simulink model "LLC_Controller"  (R2022b)
settings: Solver=FixedStepDiscrete  StartTime=0.0  StopTime=Inf  FixedStep=(20e-6)  RelTol=1e-3  EnableMultiTasking=on
undefined symbols (not defined in the file): GPTRIP1SEL, GPTRIP2SEL, SCI_A_Transmit, SCI_A_Transmit_Current_Suffix, SCI_A_Transmit_Duty_Suffix, SCI_A_Transmit_Freq_Suffix, SCI_A_Transmit_NewVRegPoint_Suffix, SCI_A_Transmit_OCPFlag_Suffix, SCI_A_Transmit_OVPFlag_Suffix, SCI_A_Transmit_PFC_Suffix, SCI_A_Transmit_SS_Suffix, SCI_A_Transmit_TBPHS_Suffix, SCI_A_Transmit_VADC_Suffix, SCI_A_Transmit_VAvg_Suffix, SCI_A_Transmit_VBAT_Suffix, SCI_A_Transmit_VBATRef_Suffix, SCI_A_Transmit_Vo_Suffix, TZ1, TZ2
libraries: c280xlib x16, c28003xlib x13, c2802xlib x8, simulink x7, c2837xDlib x3, c2000lib x1
(part 2 of 2)

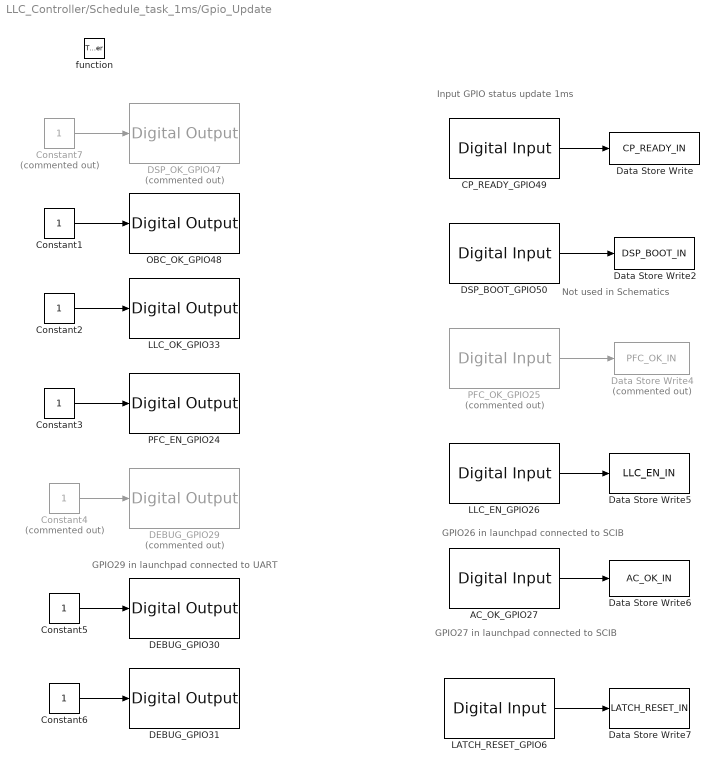
== system LLC_Controller/Schedule_task_1ms/Gpio_Update ==
  note: Not used in Schematics
  note: GPIO29 in launchpad connected to UART
  note: GPIO26 in launchpad connected to SCIB
  note: GPIO27 in launchpad connected to SCIB
  note: Input GPIO status update 1ms
  function : TriggerPort  TriggerType=function-call  VariantControl=(inherit)
  AC_OK_GPIO27 : c28003xlib/Digital Input  GPIO_Number=GPIO24~GPIO31  GPIO_Bit0=off  GPIO_Bit1=off  GPIO_Bit2=off  GPIO_Bit3=on  GPIO_Bit4=off  GPIO_Bit5=off  GPIO_Bit6=off  GPIO_Bit7=off  sampleTime=-1  dataType=auto  GPIO_Bit0_Qualification=Sync to SYSCLKOUT  GPIO_Bit1_Qualification=Sync to SYSCLKOUT  GPIO_Bit2_Qualification=Sync to SYSCLKOUT  GPIO_Bit3_Qualification=Sync to SYSCLKOUT  GPIO_Bit4_Qualification=Sync to SYSCLKOUT  GPIO_Bit5_Qualification=Sync to SYSCLKOUT  GPIO_Bit6_Qualification=Sync to SYSCLKOUT  GPIO_Bit7_Qualification=Sync to SYSCLKOUT  Qualification_Period=-1
  CP_READY_GPIO49 : c28003xlib/Digital Input  GPIO_Number=GPIO48~GPIO55  GPIO_Bit0=off  GPIO_Bit1=on  GPIO_Bit2=off  GPIO_Bit3=off  GPIO_Bit4=off  GPIO_Bit5=off  GPIO_Bit6=off  GPIO_Bit7=off  sampleTime=-1  dataType=auto  GPIO_Bit0_Qualification=Sync to SYSCLKOUT  GPIO_Bit1_Qualification=Sync to SYSCLKOUT  GPIO_Bit2_Qualification=Sync to SYSCLKOUT  GPIO_Bit3_Qualification=Sync to SYSCLKOUT  GPIO_Bit4_Qualification=Sync to SYSCLKOUT  GPIO_Bit5_Qualification=Sync to SYSCLKOUT  GPIO_Bit6_Qualification=Sync to SYSCLKOUT  GPIO_Bit7_Qualification=Sync to SYSCLKOUT  Qualification_Period=-1
  Constant{1..3,5..6} (5 alike) : Constant  OutDataTypeStr=boolean  SampleTime=-1
  Constant4 : Constant  Commented=on  OutDataTypeStr=boolean  SampleTime=-1
  Constant7 : Constant  Commented=on  OutDataTypeStr=boolean  SampleTime=-1
  DEBUG_GPIO29 : c28003xlib/Digital Output  Commented=on  GPIO_Number=GPIO24~GPIO31  GPIO_Bit0=off  GPIO_BIT0_Toggle=on  GPIO_Bit1=off  GPIO_BIT1_Toggle=on  GPIO_Bit2=off  GPIO_BIT2_Toggle=off  GPIO_Bit3=off  GPIO_BIT3_Toggle=off  GPIO_Bit4=off  GPIO_BIT4_Toggle=on  GPIO_Bit5=on  GPIO_BIT5_Toggle=on  GPIO_Bit6=off  GPIO_BIT6_Toggle=on  GPIO_Bit7=off  GPIO_BIT7_Toggle=on
  DEBUG_GPIO30 : c28003xlib/Digital Output  GPIO_Number=GPIO24~GPIO31  GPIO_Bit0=off  GPIO_BIT0_Toggle=on  GPIO_Bit1=off  GPIO_BIT1_Toggle=on  GPIO_Bit2=off  GPIO_BIT2_Toggle=off  GPIO_Bit3=off  GPIO_BIT3_Toggle=off  GPIO_Bit4=off  GPIO_BIT4_Toggle=on  GPIO_Bit5=off  GPIO_BIT5_Toggle=on  GPIO_Bit6=on  GPIO_BIT6_Toggle=on  GPIO_Bit7=off  GPIO_BIT7_Toggle=on
  DEBUG_GPIO31 : c28003xlib/Digital Output  GPIO_Number=GPIO24~GPIO31  GPIO_Bit0=off  GPIO_BIT0_Toggle=on  GPIO_Bit1=off  GPIO_BIT1_Toggle=on  GPIO_Bit2=off  GPIO_BIT2_Toggle=off  GPIO_Bit3=off  GPIO_BIT3_Toggle=off  GPIO_Bit4=off  GPIO_BIT4_Toggle=on  GPIO_Bit5=off  GPIO_BIT5_Toggle=on  GPIO_Bit6=off  GPIO_BIT6_Toggle=on  GPIO_Bit7=on  GPIO_BIT7_Toggle=on
  DSP_BOOT_GPIO50 : c28003xlib/Digital Input  GPIO_Number=GPIO48~GPIO55  GPIO_Bit0=off  GPIO_Bit1=off  GPIO_Bit2=on  GPIO_Bit3=off  GPIO_Bit4=off  GPIO_Bit5=off  GPIO_Bit6=off  GPIO_Bit7=off  sampleTime=-1  dataType=auto  GPIO_Bit0_Qualification=Sync to SYSCLKOUT  GPIO_Bit1_Qualification=Sync to SYSCLKOUT  GPIO_Bit2_Qualification=Sync to SYSCLKOUT  GPIO_Bit3_Qualification=Sync to SYSCLKOUT  GPIO_Bit4_Qualification=Sync to SYSCLKOUT  GPIO_Bit5_Qualification=Sync to SYSCLKOUT  GPIO_Bit6_Qualification=Sync to SYSCLKOUT  GPIO_Bit7_Qualification=Sync to SYSCLKOUT  Qualification_Period=-1
  DSP_OK_GPIO47 : c28003xlib/Digital Output  Commented=on  GPIO_Number=GPIO40~GPIO47  GPIO_Bit0=off  GPIO_BIT0_Toggle=on  GPIO_Bit1=off  GPIO_BIT1_Toggle=off  GPIO_Bit2=off  GPIO_BIT2_Toggle=off  GPIO_Bit3=off  GPIO_BIT3_Toggle=off  GPIO_Bit4=off  GPIO_BIT4_Toggle=on  GPIO_Bit5=off  GPIO_BIT5_Toggle=off  GPIO_Bit6=off  GPIO_BIT6_Toggle=off  GPIO_Bit7=on  GPIO_BIT7_Toggle=off
  Data Store Write : DataStoreWrite  DataStoreName=CP_READY_IN  IndexOptions=Index vector (dialog)  Indices=1  OutputSizes=1
  Data Store Write2 : DataStoreWrite  DataStoreName=DSP_BOOT_IN  IndexOptions=Index vector (dialog)  Indices=1  OutputSizes=1
  Data Store Write4 : DataStoreWrite  Commented=on  DataStoreName=PFC_OK_IN  IndexOptions=Index vector (dialog)  Indices=1  OutputSizes=1
  Data Store Write5 : DataStoreWrite  DataStoreName=LLC_EN_IN  IndexOptions=Index vector (dialog)  Indices=1  OutputSizes=1
  Data Store Write6 : DataStoreWrite  DataStoreName=AC_OK_IN  IndexOptions=Index vector (dialog)  Indices=1  OutputSizes=1
  Data Store Write7 : DataStoreWrite  DataStoreName=LATCH_RESET_IN  IndexOptions=Index vector (dialog)  Indices=1  OutputSizes=1
  LATCH_RESET_GPIO6 : c28003xlib/Digital Input  GPIO_Number=GPIO0~GPIO7  GPIO_Bit0=off  GPIO_Bit1=off  GPIO_Bit2=off  GPIO_Bit3=off  GPIO_Bit4=off  GPIO_Bit5=off  GPIO_Bit6=on  GPIO_Bit7=off  sampleTime=-1  dataType=auto  GPIO_Bit0_Qualification=Sync to SYSCLKOUT  GPIO_Bit1_Qualification=Sync to SYSCLKOUT  GPIO_Bit2_Qualification=Sync to SYSCLKOUT  GPIO_Bit3_Qualification=Sync to SYSCLKOUT  GPIO_Bit4_Qualification=Sync to SYSCLKOUT  GPIO_Bit5_Qualification=Sync to SYSCLKOUT  GPIO_Bit6_Qualification=Sync to SYSCLKOUT  GPIO_Bit7_Qualification=Sync to SYSCLKOUT  Qualification_Period=-1
  LLC_EN_GPIO26 : c28003xlib/Digital Input  GPIO_Number=GPIO24~GPIO31  GPIO_Bit0=off  GPIO_Bit1=off  GPIO_Bit2=on  GPIO_Bit3=off  GPIO_Bit4=off  GPIO_Bit5=off  GPIO_Bit6=off  GPIO_Bit7=off  sampleTime=-1  dataType=auto  GPIO_Bit0_Qualification=Sync to SYSCLKOUT  GPIO_Bit1_Qualification=Sync to SYSCLKOUT  GPIO_Bit2_Qualification=Sync to SYSCLKOUT  GPIO_Bit3_Qualification=Sync to SYSCLKOUT  GPIO_Bit4_Qualification=Sync to SYSCLKOUT  GPIO_Bit5_Qualification=Sync to SYSCLKOUT  GPIO_Bit6_Qualification=Sync to SYSCLKOUT  GPIO_Bit7_Qualification=Sync to SYSCLKOUT  Qualification_Period=-1
  LLC_OK_GPIO33 : c28003xlib/Digital Output  GPIO_Number=GPIO32~GPIO39  GPIO_Bit0=off  GPIO_BIT0_Toggle=off  GPIO_Bit1=on  GPIO_BIT1_Toggle=on  GPIO_Bit2=off  GPIO_BIT2_Toggle=off  GPIO_Bit3=off  GPIO_BIT3_Toggle=off  GPIO_Bit4=off  GPIO_BIT4_Toggle=on  GPIO_Bit5=off  GPIO_BIT5_Toggle=off  GPIO_Bit6=off  GPIO_BIT6_Toggle=off  GPIO_Bit7=off  GPIO_BIT7_Toggle=off
  OBC_OK_GPIO48 : c28003xlib/Digital Output  GPIO_Number=GPIO48~GPIO55  GPIO_Bit0=on  GPIO_BIT0_Toggle=on  GPIO_Bit1=off  GPIO_BIT1_Toggle=off  GPIO_Bit2=off  GPIO_BIT2_Toggle=off  GPIO_Bit3=off  GPIO_BIT3_Toggle=off  GPIO_Bit4=off  GPIO_BIT4_Toggle=on  GPIO_Bit5=off  GPIO_BIT5_Toggle=off  GPIO_Bit6=off  GPIO_BIT6_Toggle=off  GPIO_Bit7=off  GPIO_BIT7_Toggle=off
  PFC_EN_GPIO24 : c28003xlib/Digital Output  GPIO_Number=GPIO24~GPIO31  GPIO_Bit0=on  GPIO_BIT0_Toggle=on  GPIO_Bit1=off  GPIO_BIT1_Toggle=on  GPIO_Bit2=off  GPIO_BIT2_Toggle=off  GPIO_Bit3=off  GPIO_BIT3_Toggle=off  GPIO_Bit4=off  GPIO_BIT4_Toggle=on  GPIO_Bit5=off  GPIO_BIT5_Toggle=off  GPIO_Bit6=off  GPIO_BIT6_Toggle=off  GPIO_Bit7=off  GPIO_BIT7_Toggle=off
  PFC_OK_GPIO25 : c28003xlib/Digital Input  Commented=on  GPIO_Number=GPIO24~GPIO31  GPIO_Bit0=off  GPIO_Bit1=on  GPIO_Bit2=off  GPIO_Bit3=off  GPIO_Bit4=off  GPIO_Bit5=off  GPIO_Bit6=off  GPIO_Bit7=off  sampleTime=-1  dataType=auto  GPIO_Bit0_Qualification=Sync to SYSCLKOUT  GPIO_Bit1_Qualification=Sync to SYSCLKOUT  GPIO_Bit2_Qualification=Sync to SYSCLKOUT  GPIO_Bit3_Qualification=Sync to SYSCLKOUT  GPIO_Bit4_Qualification=Sync to SYSCLKOUT  GPIO_Bit5_Qualification=Sync to SYSCLKOUT  GPIO_Bit6_Qualification=Sync to SYSCLKOUT  GPIO_Bit7_Qualification=Sync to SYSCLKOUT  Qualification_Period=-1
  wires:
  Constant1/1 -> OBC_OK_GPIO48/1
  Constant2/1 -> LLC_OK_GPIO33/1
  AC_OK_GPIO27/1 -> Data Store Write6/1
  LATCH_RESET_GPIO6/1 -> Data Store Write7/1
  PFC_OK_GPIO25/1 -> Data Store Write4/1
  Constant4/1 -> DEBUG_GPIO29/1
  CP_READY_GPIO49/1 -> Data Store Write/1
  LLC_EN_GPIO26/1 -> Data Store Write5/1
  DSP_BOOT_GPIO50/1 -> Data Store Write2/1
  Constant6/1 -> DEBUG_GPIO31/1
  Constant3/1 -> PFC_EN_GPIO24/1
  Constant5/1 -> DEBUG_GPIO30/1
  Constant7/1 -> DSP_OK_GPIO47/1

== system LLC_Controller/State_Machine/LLC_STATEFLOW/SSvoltage ==
  f : TriggerPort  TriggerType=function-call  VariantControl=(inherit)
      settings: CopyFcn=Stateflow.SLINSF.SimulinkMan.removeBlockPreDeleteFcn  PreDeleteFcn=Stateflow.SLINSF.SimulinkMan.unsafePredeleteFcn
  Chart1 : Stateflow chart  TreatAsAtomicUnit=on
  Constant1 : Constant  OutDataTypeStr=double  SampleTime=Inf
  wires:
  Constant1/1 -> Chart1/1(VBAT_Ref)

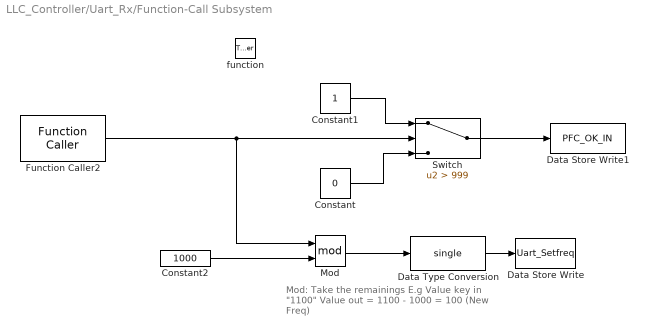
== system LLC_Controller/Uart_Rx/Function-Call Subsystem ==
  note: Mod: Take the remainings
      | E.g
      | Value key in "1100"
      | Value out = 1100 - 1000 = 100 (New Freq)
  function : TriggerPort  TriggerType=function-call  VariantControl=(inherit)
  Constant : Constant  Value=0
  Constant1 : Constant
  Constant2 : Constant  Value=1000
  Data Store Write : DataStoreWrite  DataStoreName=Uart_Setfreq  IndexOptions=Index vector (dialog)  Indices=1  OutputSizes=1
  Data Store Write1 : DataStoreWrite  DataStoreName=PFC_OK_IN  IndexOptions=Index vector (dialog)  Indices=1  OutputSizes=1
  Data Type Conversion : DataTypeConversion  OutDataTypeStr=single  SaturateOnIntegerOverflow=off  RndMeth=Floor
  Function Caller2 : FunctionCaller  FunctionPrototype=y = SCI_Receive()  InputArgumentSpecifications=<Enter example>  OutputArgumentSpecifications=<Enter example>
  Mod : Math  Operator=mod
  Switch : Switch  Criteria=u2 > Threshold  Threshold=999  SaturateOnIntegerOverflow=off  InputSameDT=off
  wires:
  Switch/1 -> Data Store Write1/1
  Function Caller2/1 -> Mod/1, Switch/2
  Constant/1 -> Switch/3
  Constant1/1 -> Switch/1
  Mod/1 -> Data Type Conversion/1
  Constant2/1 -> Mod/2
  Data Type Conversion/1 -> Data Store Write/1

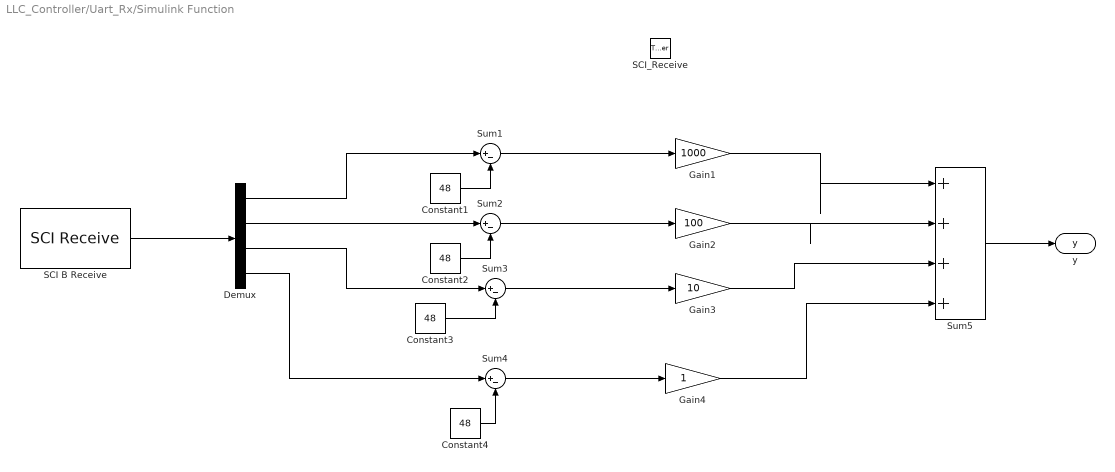
== system LLC_Controller/Uart_Rx/Simulink Function ==
  SCI_Receive : TriggerPort  TriggerType=function-call  IsSimulinkFunction=on  FunctionName=SCI_Receive  FunctionVisibility=scoped  VariantControl=(inherit)
  Constant{1..4} (4 alike) : Constant  Value=48
  Demux : Demux
  Gain1 : Gain  Gain=1000
  Gain2 : Gain  Gain=100
  Gain3 : Gain  Gain=10
  Gain4 : Gain
  SCI B Receive : c280xlib/SCI Receive  Priority=2  sciModule=A  dataHead=''  headerCheckMaxCount=16  dataTail=''  dataType=uint8  dataLenOptions=Length via dialog  dataDim=4  maxDataLength=100  initValue=0  errOption=Output custom value  errValue=0  sampleTime=-1  blockingMode=on  timeOut=0.01944  outputStatus=off
      settings: LibrarySourceBlock=c2806xlib/SCI Receive
  Sum{1..4} (4 alike) : Sum  Inputs=|+-
  Sum5 : Sum  Inputs=|++++  AccumDataTypeStr=double  OutDataTypeStr=double
  y : ArgOut  DisableCoverage=on  ArgumentName=y
  wires:
  Gain2/1 -> Sum5/2
  Gain3/1 -> Sum5/3
  Constant3/1 -> Sum3/2
  Sum4/1 -> Gain4/1
  Constant2/1 -> Sum2/2
  Sum2/1 -> Gain2/1
  SCI B Receive/1 -> Demux/1
  Constant4/1 -> Sum4/2
  Sum3/1 -> Gain3/1
  Sum5/1 -> y/1
  Demux/4 -> Sum4/1
  Demux/3 -> Sum3/1
  Demux/2 -> Sum2/1
  Constant1/1 -> Sum1/2
  Demux/1 -> Sum1/1
  Gain4/1 -> Sum5/4
  Gain1/1 -> Sum5/1
  Sum1/1 -> Gain1/1

== system LLC_Controller/LLC Control/LLC_On_Off_Control/Subsystem_llc_off ==
  Action Port : ActionPort  ActionPortLabel=else
  Constant : Constant  OutDataTypeStr=boolean
  Data Store Write : DataStoreWrite  DataStoreName=LLC_Clr_tz  IndexOptions=Index vector (dialog)  Indices=1  OutputSizes=1
  PWM_LLC_OFF : Subsystem  mask(System Outputs){ShowInLibBrowser=0}
      mask prompts: ShowInLibBrowser "Simulink:masks:CustCodeMaskParam1_MP"
      settings: CopyFcn=cccopyfcn(gcb)  OpenFcn=ccopenfcn('System Outputs Function')
      mask Help: eval('feval(''rtwprivate'',''rtwhelpview'',''rtw_sys_outputs_block'')');
      mask DialogControl ShowInLibBrowser Prompt: Mask Parameter 1:
      mask Display: disp('System\nOutputs');
  wires:
  Constant/1 -> Data Store Write/1

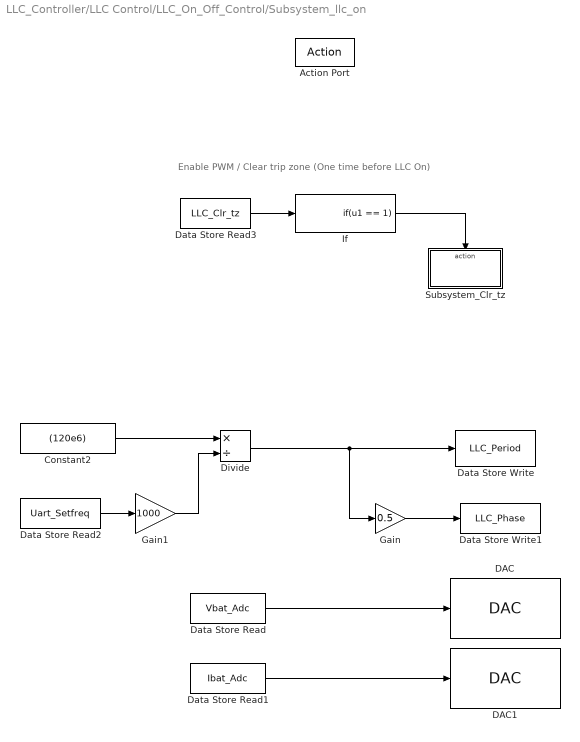
== system LLC_Controller/LLC Control/LLC_On_Off_Control/Subsystem_llc_on ==
  note: Enable PWM / Clear trip zone (One time before LLC On)
  Action Port : ActionPort  ActionPortLabel=if(u1 == 1)
  Constant2 : Constant  Value=(120e6)  OutDataTypeStr=single  SampleTime=-1
  DAC : c2837xDlib/DAC  channel=A  saturate=on
      settings: LibrarySourceBlock=c28003xlib/DAC
  DAC1 : c2837xDlib/DAC  channel=B  saturate=on
      settings: LibrarySourceBlock=c28003xlib/DAC
  Data Store Read : DataStoreRead  DataStoreName=Vbat_Adc  IndexOptions=Index vector (dialog)  Indices=1  OutputSizes=1
  Data Store Read1 : DataStoreRead  DataStoreName=Ibat_Adc  IndexOptions=Index vector (dialog)  Indices=1  OutputSizes=1
  Data Store Read2 : DataStoreRead  DataStoreName=Uart_Setfreq  IndexOptions=Index vector (dialog)  Indices=1  OutputSizes=1
  Data Store Read3 : DataStoreRead  DataStoreName=LLC_Clr_tz  IndexOptions=Index vector (dialog)  Indices=1  OutputSizes=1
  Data Store Write : DataStoreWrite  DataStoreName=LLC_Period  IndexOptions=Index vector (dialog)  Indices=1  OutputSizes=1
  Data Store Write1 : DataStoreWrite  DataStoreName=LLC_Phase  IndexOptions=Index vector (dialog)  Indices=1  OutputSizes=1
  Divide : Product  Inputs=*/  OutDataTypeStr=single
  Gain : Gain  Gain=0.5  OutDataTypeStr=single
  Gain1 : Gain  Gain=1000  OutDataTypeStr=single
  If : If  IfExpression=u1 == 1  ShowElse=off
  Subsystem_Clr_tz : Subsystem  TreatAsAtomicUnit=on
  wires:
  If/1 -> Subsystem_Clr_tz/Action
  Data Store Read3/1 -> If/1
  Divide/1 -> Gain/1, Data Store Write/1
  Gain/1 -> Data Store Write1/1
  Data Store Read/1 -> DAC/1
  Data Store Read1/1 -> DAC1/1
  Constant2/1 -> Divide/1
  Gain1/1 -> Divide/2
  Data Store Read2/1 -> Gain1/1

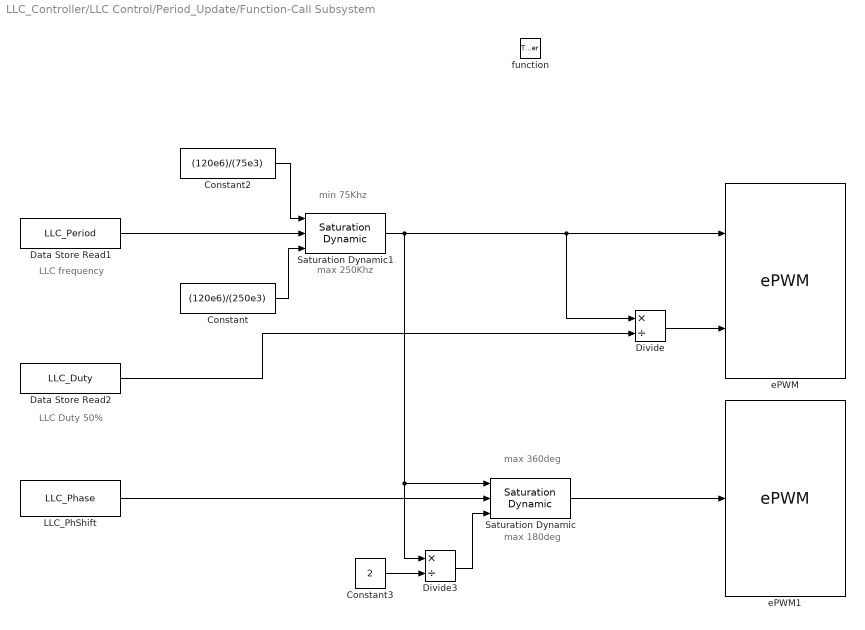
== system LLC_Controller/LLC Control/Period_Update/Function-Call Subsystem ==
  note: LLC frequency
  note: LLC Duty 50%
  note: max 180deg
  note: max 360deg
  note: min 75Khz
  note: max 250Khz
  function : TriggerPort  TriggerType=function-call  VariantControl=(inherit)
  Constant : Constant  Value=(120e6)/(250e3)  OutDataTypeStr=single  SampleTime=-1
  Constant2 : Constant  Value=(120e6)/(75e3)  OutDataTypeStr=single  SampleTime=-1
  Constant3 : Constant  Value=2  OutDataTypeStr=single  SampleTime=-1
  Data Store Read1 : DataStoreRead  DataStoreName=LLC_Period  IndexOptions=Index vector (dialog)  Indices=1  OutputSizes=1
  Data Store Read2 : DataStoreRead  DataStoreName=LLC_Duty  IndexOptions=Index vector (dialog)  Indices=1  OutputSizes=1
  Divide : Product  Inputs=*/
  Divide3 : Product  Inputs=*/
  LLC_PhShift : DataStoreRead  DataStoreName=LLC_Phase  IndexOptions=Index vector (dialog)  Indices=1  OutputSizes=1
  Saturation Dynamic : simulink/Discontinuities/Saturation Dynamic  OutMin=[]  OutMax=[]  OutDataTypeStr=Inherit: Same as second input  OutDataType=fixdt(1, 16)  OutScaling=2^-10  DoSatur=off
  Saturation Dynamic1 : simulink/Discontinuities/Saturation Dynamic  OutMin=[]  OutMax=[]  OutDataTypeStr=Inherit: Same as second input  OutDataType=fixdt(1, 16)  OutScaling=2^-10  DoSatur=off
  ePWM : c2802xlib/ePWM  PwmType=C2000_Type4_F28002x  useModule=ePWM5  ePWMxLINKTBPRD=Not Linked  periodUnits=Clock cycles  timerSource=Input port  timerPeriod_clk=600  timerPeriod_sec=0.0001  tbshadow=Counter equals to zero  countingMode=Up  phaseActiveEnable=Disable  phaseDirection=Count down after sync  phaseActive=0  synchronizationEnable=off  dcaevt1Sync=off  dcbevt1Sync=off  synchronizationOption=Counter equals to zero (CTR=Zero)  dcbevt1SyncOut=off  dcaevt1SyncOut=off  cmpdSyncOut=off  cmpcSyncOut=off  cmpbSyncOut=off  zeroSyncOut=on  swfSyncOut=off  perSynchronizationOption=Counter equals to period (CTR=PRD)  clockPrescale=1  HSclockPrescale=1  enswap=off  ePWMxAStatus=on  ePWMxAactionLogic1=Set  ePWMxAactionLogic2=Do nothing  ePWMxAactionLogic3=Clear  ePWMxAactionLogic4=Do nothing  ePWMxAactionLogic5=Do nothing  ePWMxAactionLogic6=Do nothing  ePWMxACSFenable=off  ePWMxACSFvalue=Forcing disable  ePWMxASFreload=Zero  ePWMxBStatus=on  ePWMxBactionLogic1=Clear  ePWMxBactionLogic2=Do nothing  ePWMxBactionLogic3=Set  ePWMxBactionLogic4=Do nothing  ePWMxBactionLogic5=Do nothing  ePWMxBactionLogic6=Set  ePWMxBCSFenable=off  ePWMxBCSFvalue=Forcing disable  ePWMxBSFreload=Zero  ePWNxBOutWay=off  ePWMxLINKCMPA=Not Linked  CMPAUnits=Clock cycles  CMPASource=Input port  CMPAValue_per=50  CMPAValue_clk=298  enCMPAshadow=Counter equals to zero (CTR=Zero)  ePWMxLINKCMPB=Not Linked  CMPBUnits=Clock cycles  CMPBSource=Specify via dialog  CMPBValue_per=50  CMPBValue_clk=0  enCMPBshadow=Counter equals to zero (CTR=Zero)  ePWMxLINKCMPC=Not Linked  CMPCUnits=Clock cycles  CMPCSource=Specify via dialog  CMPCValue_per=50  CMPCValue_clk=32000  enCMPCshadow=Counter equals to zero (CTR=Zero)  ePWMxLINKCMPD=Not Linked  CMPDUnits=Percentages  CMPDSource=Specify via dialog  CMPDValue_per=50  CMPDValue_clk=32000  enCMPDshadow=Counter equals to zero (CTR=Zero)  enableDBePWMxA=on  enableDBePWMxB=on  enhalfcycle=off  DBpolarity=Active high complementary (AHC)  DBedgeDelay=Positive  DBSource_ePWMxA=ePWMxA  DBSource_ePWMxB=ePWMxA  DBPeriodUnits=Seconds  DBperiodSource=Specify via dialog  REDperiod=0  FEDperiod=0  REDperiod_sec=250e-9  FEDperiod_sec=250e-9  LoadModeDBRED=Counter equals to zero (CTR=ZERO)  LoadModeDBFED=Counter equals to zero (CTR=ZERO)  adcstartModuleA=off  adcrequestEventA=First event  adcstartEventA=Counter equals to zero (CTR=Zero)  adcstartEventA_type2=Counter equals to zero (CTR=Zero)  adcstartModuleB=off  adcrequestEventB=First event  adcstartEventB=Counter equals to zero (CTR=Zero)  adcstartEventB_type2=Counter equals to zero (CTR=Zero)  intEn=off  intPrd=First event  intSel=Counter equals to zero (CTR=Zero)  intSel_type2=Counter equals to zero (CTR=Zero)  hrpe=off  enHRPWM=off  HRPWM_LoadMode=Counter equals to zero (CTR=ZERO)  HRPWM_CTLMode=Duty or Period control mode  HRPWM_EDGMode=Both edge  hrpeb=off  enHRPWMB=off  HRPWM_LoadModeB=Counter equals to zero (CTR=ZERO)  HRPWM_CTLModeB=Duty or Period control mode  HRPWM_EDGModeB=Both edge  enHRDBRED=off  enHRDBFED=off  enSFO=on  enautoconv=on  chopperEnable=off  chopperFrequency=1  chopperFirstwidth=1  chopperDuty=12.5%  tripZonesource=Specify via dialog  tzselOSHT1=off  tzselOSHT2=off  tzselOSHT3=off  tzselOSHDCAEV1=off  tzselOSHDCBEV1=off  tzselCBC1=off  tzselCBC2=off  tzselCBC3=off  tzselCBCDCAEV2=off  tzselCBCDCBEV2=off  tzselOSHT4=off  tzselOSHT5=off  tzselOSHT6=off  tzselCBC4=off  tzselCBC5=off  tzselCBC6=off  enTzOstIntr=off  enTzCbcIntr=off  enTzDCAEVT1Intr=off  enTzDCAEVT2Intr=off  enTzDCBEVT1Intr=off  enTzDCBEVT2Intr=off  ePWMxAforced=Low  ePWMxBforced=Low  DCAEVT1forced=No action  DCBEVT1forced=No action  DCAEVT2forced=No action  DCBEVT2forced=No action  dcah=Trip Zone 1 input (TZ1)  dcal=Trip Zone 1 input (TZ1)  dcbh=Trip Zone 1 input (TZ1)  dcbl=Trip Zone 1 input (TZ1)  dcah_type2=GPTRIP4SEL  dcal_type2=GPTRIP1SEL/(TZ1)  dcbh_type2=GPTRIP4SEL  dcbl_type2=GPTRIP2SEL/(TZ2)  gendcaevt1=DCAH=high and DCAL=don't care  gendcaevt2=Event disabled  gendcbevt1=DCBH=high and DCBL=don't care  gendcbevt2=Event disabled  dcaevt1src=DCAEVT1 with async  dcaevt2src=DCAEVT2 with sync  dcbevt1src=DCBEVT1 with async  dcbevt2src=DCBEVT2 with sync  pulsesel=Counter equals to zero (CTR=Zero)  blankinv=off  blankoffset=0  blankwidth=0  evsrcsel=Filtered version of DCAEVT1 (DCAEVT1FILT)  encape=off
  ePWM1 : c2802xlib/ePWM  PwmType=C2000_Type4_F28002x  useModule=ePWM7  ePWMxLINKTBPRD=ePWM5  periodUnits=Clock cycles  timerSource=Specify via dialog  timerPeriod_clk=600  timerPeriod_sec=0.0001  tbshadow=Counter equals to zero  countingMode=Up  phaseActiveEnable=Set counter to phase value specified via input port  phaseDirection=Count down after sync  phaseActive=0  synchronizationEnable=off  dcaevt1Sync=off  dcbevt1Sync=off  synchronizationOption=Counter equals to zero (CTR=Zero)  dcbevt1SyncOut=off  dcaevt1SyncOut=off  cmpdSyncOut=off  cmpcSyncOut=off  cmpbSyncOut=off  zeroSyncOut=on  swfSyncOut=off  perSynchronizationOption=Counter equals to zero (CTR=Zero)  clockPrescale=1  HSclockPrescale=1  enswap=off  ePWMxAStatus=on  ePWMxAactionLogic1=Set  ePWMxAactionLogic2=Do nothing  ePWMxAactionLogic3=Clear  ePWMxAactionLogic4=Do nothing  ePWMxAactionLogic5=Do nothing  ePWMxAactionLogic6=Do nothing  ePWMxACSFenable=off  ePWMxACSFvalue=Forcing disable  ePWMxASFreload=Zero  ePWMxBStatus=on  ePWMxBactionLogic1=Clear  ePWMxBactionLogic2=Do nothing  ePWMxBactionLogic3=Set  ePWMxBactionLogic4=Do nothing  ePWMxBactionLogic5=Do nothing  ePWMxBactionLogic6=Set  ePWMxBCSFenable=off  ePWMxBCSFvalue=Forcing disable  ePWMxBSFreload=Zero  ePWNxBOutWay=off  ePWMxLINKCMPA=ePWM5  CMPAUnits=Clock cycles  CMPASource=Specify via dialog  CMPAValue_per=50  CMPAValue_clk=298  enCMPAshadow=Counter equals to zero (CTR=Zero)  ePWMxLINKCMPB=Not Linked  CMPBUnits=Clock cycles  CMPBSource=Specify via dialog  CMPBValue_per=50  CMPBValue_clk=0  enCMPBshadow=Counter equals to zero (CTR=Zero)  ePWMxLINKCMPC=Not Linked  CMPCUnits=Clock cycles  CMPCSource=Specify via dialog  CMPCValue_per=50  CMPCValue_clk=32000  enCMPCshadow=Counter equals to zero (CTR=Zero)  ePWMxLINKCMPD=Not Linked  CMPDUnits=Percentages  CMPDSource=Specify via dialog  CMPDValue_per=50  CMPDValue_clk=32000  enCMPDshadow=Counter equals to zero (CTR=Zero)  enableDBePWMxA=on  enableDBePWMxB=on  enhalfcycle=off  DBpolarity=Active high complementary (AHC)  DBedgeDelay=Positive  DBSource_ePWMxA=ePWMxA  DBSource_ePWMxB=ePWMxA  DBPeriodUnits=Seconds  DBperiodSource=Specify via dialog  REDperiod=0  FEDperiod=0  REDperiod_sec=250e-9  FEDperiod_sec=250e-9  LoadModeDBRED=Counter equals to zero (CTR=ZERO)  LoadModeDBFED=Counter equals to zero (CTR=ZERO)  adcstartModuleA=off  adcrequestEventA=First event  adcstartEventA=Counter equals to zero (CTR=Zero)  adcstartEventA_type2=Counter equals to zero (CTR=Zero)  adcstartModuleB=off  adcrequestEventB=First event  adcstartEventB=Counter equals to zero (CTR=Zero)  adcstartEventB_type2=Counter equals to zero (CTR=Zero)  intEn=off  intPrd=First event  intSel=Counter equals to zero (CTR=Zero)  intSel_type2=Counter equals to zero (CTR=Zero)  hrpe=off  enHRPWM=off  HRPWM_LoadMode=Counter equals to period (CTR=PRD)  HRPWM_CTLMode=Duty or Period control mode  HRPWM_EDGMode=Both edge  hrpeb=off  enHRPWMB=off  HRPWM_LoadModeB=Counter equals to zero (CTR=ZERO)  HRPWM_CTLModeB=Duty or Period control mode  HRPWM_EDGModeB=Both edge  enHRDBRED=off  enHRDBFED=off  enSFO=on  enautoconv=on  chopperEnable=off  chopperFrequency=1  chopperFirstwidth=1  chopperDuty=12.5%  tripZonesource=Specify via dialog  tzselOSHT1=off  tzselOSHT2=off  tzselOSHT3=off  tzselOSHDCAEV1=off  tzselOSHDCBEV1=off  tzselCBC1=off  tzselCBC2=off  tzselCBC3=off  tzselCBCDCAEV2=off  tzselCBCDCBEV2=off  tzselOSHT4=off  tzselOSHT5=off  tzselOSHT6=off  tzselCBC4=off  tzselCBC5=off  tzselCBC6=off  enTzOstIntr=off  enTzCbcIntr=off  enTzDCAEVT1Intr=off  enTzDCAEVT2Intr=off  enTzDCBEVT1Intr=off  enTzDCBEVT2Intr=off  ePWMxAforced=Low  ePWMxBforced=Low  DCAEVT1forced=No action  DCBEVT1forced=No action  DCAEVT2forced=No action  DCBEVT2forced=No action  dcah=Trip Zone 1 input (TZ1)  dcal=Trip Zone 1 input (TZ1)  dcbh=Trip Zone 1 input (TZ1)  dcbl=Trip Zone 1 input (TZ1)  dcah_type2=GPTRIP4SEL  dcal_type2=GPTRIP2SEL/(TZ2)  dcbh_type2=GPTRIP4SEL  dcbl_type2=GPTRIP2SEL/(TZ2)  gendcaevt1=DCAH=high and DCAL=don't care  gendcaevt2=Event disabled  gendcbevt1=DCBH=high and DCBL=don't care  gendcbevt2=Event disabled  dcaevt1src=DCAEVT1 with async  dcaevt2src=DCAEVT2 with sync  dcbevt1src=DCBEVT1 with async  dcbevt2src=DCBEVT2 with sync  pulsesel=Counter equals to zero (CTR=Zero)  blankinv=off  blankoffset=0  blankwidth=0  evsrcsel=Filtered version of DCAEVT1 (DCAEVT1FILT)  encape=off
  wires:
  Saturation Dynamic/1 -> ePWM1/1
  Divide/1 -> ePWM/2
  Data Store Read2/1 -> Divide/2
  Constant/1 -> Saturation Dynamic1/3
  Saturation Dynamic1/1 -> Divide3/1, Saturation Dynamic/1, Divide/1, ePWM/1
  Constant2/1 -> Saturation Dynamic1/1
  Divide3/1 -> Saturation Dynamic/3
  Constant3/1 -> Divide3/2
  LLC_PhShift/1 -> Saturation Dynamic/2
  Data Store Read1/1 -> Saturation Dynamic1/2

== system LLC_Controller/LLC Control/Period_Update/Function-Call Subsystem1 ==
  function : TriggerPort  TriggerType=function-call  VariantControl=(inherit)
  PWM_UPDATE : Subsystem  mask(System Outputs){ShowInLibBrowser=0}
      mask prompts: ShowInLibBrowser "Simulink:masks:CustCodeMaskParam1_MP"
      settings: CopyFcn=cccopyfcn(gcb)  OpenFcn=ccopenfcn('System Outputs Function')
      mask Help: eval('feval(''rtwprivate'',''rtwhelpview'',''rtw_sys_outputs_block'')');
      mask DialogControl ShowInLibBrowser Prompt: Mask Parameter 1:
      mask Display: disp('System\nOutputs');

== system LLC_Controller/LLC Control/LLC_On_Off_Control/Subsystem_llc_off/PWM_LLC_OFF ==

== system LLC_Controller/LLC Control/LLC_On_Off_Control/Subsystem_llc_on/Subsystem_Clr_tz ==
  Action Port : ActionPort  ActionPortLabel=if(u1 == 1)
  CMPSS : c2837xDlib/CMPSS  Module=CMPSS2_COMPH  NegativeInput=Internal DAC  DacValueSourceSel=DAC module  DacValueVia=Input port  DACHValue=0  DACLValue=0  RampMaxRefVal=0  RampDecVal=0  RampDelayVal=0  EnableLatchOut=off  EnableLatchClear=off  SampleTime=0.1
      settings: LibrarySourceBlock=c28003xlib/CMPSS
  Constant : Constant  Value=0  OutDataTypeStr=boolean
  Constant1 : Constant  Value=2500  SampleTime=-1
  Data Store Write : DataStoreWrite  DataStoreName=LLC_Clr_tz  IndexOptions=Index vector (dialog)  Indices=1  OutputSizes=1
  PWM_LLC_ON : Subsystem  mask(System Outputs){ShowInLibBrowser=0}
      mask prompts: ShowInLibBrowser "Simulink:masks:CustCodeMaskParam1_MP"
      settings: CopyFcn=cccopyfcn(gcb)  OpenFcn=ccopenfcn('System Outputs Function')
      mask Help: eval('feval(''rtwprivate'',''rtwhelpview'',''rtw_sys_outputs_block'')');
      mask DialogControl ShowInLibBrowser Prompt: Mask Parameter 1:
      mask Display: disp('System\nOutputs');
  wires:
  Constant/1 -> Data Store Write/1
  Constant1/1 -> CMPSS/1

== system LLC_Controller/LLC Control/Period_Update/Function-Call Subsystem1/PWM_UPDATE ==

== system LLC_Controller/LLC Control/LLC_On_Off_Control/Subsystem_llc_on/Subsystem_Clr_tz/PWM_LLC_ON ==

== matlab function LLC_Controller/Schedule_task_100ms/SCI_A_Transmit_function2/MATLAB Function ==
  data: Main_number input; Digit_5 output; Divider input; Digit_4 output; Digit_3 output; Digit_2 output; Digit_1 output
function [Digit_5,Digit_4,Digit_3,Digit_2,Digit_1]  = fcn(Main_number,Divider)

R_Digit_5 = rem(Main_number,Divider);
Q_Digit_5 = (Main_number-R_Digit_5)/Divider;
Digit_5 = uint8(Q_Digit_5);
%Digit_5 done

R_Digit_4 = rem(R_Digit_5,Divider/10);
Q_Digit_4 = (R_Digit_5-R_Digit_4)/(Divider/10);
Digit_4 = uint8(Q_Digit_4);
%Digit_4 done

R_Digit_3 = rem(R_Digit_4,Divider/100);
Q_Digit_3 = (R_Digit_4-R_Digit_3)/(Divider/100);
Digit_3 = uint8(Q_Digit_3);
%Digit_3 done

R_Digit_2 = rem(R_Digit_3,Divider/1000);
Q_Digit_2 = (R_Digit_3-R_Digit_2)/(Divider/1000);
Digit_2 = uint8(Q_Digit_2);
%Digit_2 done

R_Digit_1 = rem(R_Digit_2,Divider/10000);
Q_Digit_1 = (R_Digit_2-R_Digit_1)/(Divider/10000);
Digit_1 = uint8(Q_Digit_1);
%Digit_1 done
end

== stateflow chart LLC_Controller/State_Machine/LLC_STATEFLOW/SSvoltage/Chart1 ==
  note: Verror = Vbulk_Ref_ADC_adjusted - Vbulk_ADC;
  note: Local variables
      | VbusRefTemp
      | SoftStartCnt
  (default) -> (junction 47)
  (junction 47) -> (junction 50) [order 2]
  (junction 50) -> (junction 52) : {
      | %First_Pass=1;
      | %Soft_Start=1;
      | %SoftStartCnt=1;
      | %Debug=1;
      | }
  (junction 47) -> (junction 5) [order 1] : [pfc_ok]
  (junction 5) -> (junction 7) [order 1] : [First_Pass]
  (junction 5) -> (junction 15) [order 2] : [Soft_Start]
  (junction 15) -> (junction 18) [order 1] : [SoftStartCnt>30]
      | %% 1 count = 0.2ms (5kHz)
      | %% 10 counts = 2ms
  (junction 18) -> (junction 23) [order 2] : %{Debug=Vbulk_Ref_ADC_adjusted;}
  (junction 23) -> (junction 31) : %{Debug=6;}
  (junction 31) -> (junction 55) [order 1] : [abs(VBAT_Ref_adjusted - VBAT_Ref)<0.9]
  (junction 7) -> (junction 10) : {
      | VBAT_Ref_adjusted = VBAT_Value/RegulationPoint;
      | %Vbulk_Ref_ADC_adjusted = Vbulk_Ref_ADC;
      | First_Pass = 0;
      | %Debug=2;
      |
      | }
  (junction 5) -> (junction 38) [order 3] : {
      | SoftStart_OK = 1;
      | %Debug=3;
      | %Vbulk_Ref_ADC_adjusted=Vbulk_Ref_ADC;
      |
      | }
  (junction 15) -> (junction 20) [order 2] : {
      | SoftStartCnt = SoftStartCnt + 1;
      | %Debug=4;
      | }
      | %% incerase the counter first.
  (junction 18) -> (junction 64) [order 1] : [VBAT_Ref_adjusted < VBAT_Ref]
      | {VBAT_Ref_adjusted = VBAT_Ref_adjusted + 0.1;}
      | %% Increase the reference voltage
  (junction 23) -> (junction 26) [commented out] : [VBAT_Ref_adjusted > VBAT_Ref]
      | {VBAT_Ref_adjusted = VBAT_Ref_adjusted - 0.1;
      | }
      | %% Reduce the reference voltage
  (junction 31) -> (junction 33) [order 2] : {
      | Soft_Start=0;
      | SoftStartCnt=0;
      | %Debug=7;
      | VBAT_Ref_adjusted=VBAT_Ref;
      | }
      | %% End soft start
  (junction 55) -> (junction 57) : {
      | Soft_Start=0;
      | SoftStartCnt=0;
      | VBAT_Ref_adjusted=VBAT_Ref;
      | %Debug=8;
      | }
  (junction 64) -> (junction 28) [order 2]
  (junction 64) -> (junction 28) [order 1] : [VBAT_Ref_adjusted < (VBAT_Value/RegulationPoint)]
      | {VBAT_Ref_adjusted = (VBAT_Value/RegulationPoint) ;}
      | %% Increase the reference voltage
  (junction 52) -> (junction 10)
  (junction 10) -> (junction 38)
  (junction 26) -> (junction 28)
  (junction 33) -> (junction 26)
  (junction 57) -> (junction 33)
  (junction 20) -> (junction 38)
  (junction 28) -> (junction 20)
  data: VbusRefTemp local =0; SoftStartCnt local =0; VBAT_Ref input double; Vbulk_Ref_ADC_Hard_Value local =0; First_Pass1 local; First_Pass local =1; Soft_Start local =1

== stateflow chart LLC_Controller/State_Machine/LLC_STATEFLOW ==
  state OFF_MODE
    entry:
    llc_on = 0;
  state STARTUP_MODE
    entry: llc_on = 1;
    during:
    %%add softstart%%
  state llcControlLoopwithSS(ref_calib,fb) [function] [commented out]
    note: SOFT START
    note: PFM
    note: PSPWM
    note: BURST
    (default) -> (junction 31) [commented out] : //{fbk = fb;
        | //ref = ref_calib;}
    (junction 31) -> (junction 32) [commented out] : [!eoss_llc1]{mode = 3;}
    (junction 31) -> (junction 39) [commented out]
    (junction 32) -> (junction 33) [commented out] : {diff = ref_calib - fb;}
    (junction 33) -> (junction 36) [commented out] : [diff > 11]
    (junction 33) -> (junction 35) [commented out]
    (junction 33) -> (junction 34) [commented out] : [diff < -11]
    (junction 36) -> (junction 37) [commented out] : {ref = fb + 11;
        | eoss_llc1 = 0;}
    (junction 35) -> (junction 37) [commented out] : {ref = ref_calib;
        | eoss_llc1 = 1;}
    (junction 34) -> (junction 37) [commented out] : {ref = fb - 11;
        | eoss_llc1 = 0;}
    (junction 37) -> (junction 42) [commented out]
    (junction 39) -> (junction 42) [commented out]
    (junction 39) -> (junction 38) [commented out]
    (junction 39) -> (junction 40) [commented out] : [(llc1_ts_tbctr>=pfm_integ_min) && (llc1_ps<=pspwm_integ_min) && (llc1_burstduty == 100)]
    (junction 40) -> (junction 41) [commented out] : {llc1_ts_tbctr = SSvoltage(ref, fb); mode = 2;}
    (junction 38) -> (junction 48) [commented out] : [(llc1_ts_tbctr<=pfm_integ_min) && (llc1_ps>=pspwm_integ_max)]
    (junction 39) -> (junction 43) [commented out]
    (junction 41) -> (junction 42) [commented out]
    (junction 47) -> (junction 42) [commented out]
    (junction 42) -> (junction 50) [commented out]
    (junction 43) -> (junction 44) [commented out] : [(llc1_ts_tbctr<=pfm_integ_min) && (llc1_burstduty == 100)]
    (junction 44) -> (junction 45) [commented out] : [(llc1_ps<=pspwm_integ_min) && (mode == 2 )]
    (junction 46) -> (junction 45) [commented out] : [(llc1_ps >= pspwm_integ_max) && (mode ==0)]
    (junction 46) -> (junction 45) [commented out] : [(llc1_ps > pspwm_integ_min) && (llc1_ps < pspwm_integ_max) && (mode ==1)]
    (junction 44) -> (junction 46) [commented out]
    (junction 45) -> (junction 47) [commented out] : {llc1_ps = pspwmLlc1(ref, fb); mode = 1;}
    (junction 48) -> (junction 49) [commented out]
    (junction 49) -> (junction 50) [commented out] : {llc1_burstduty = burstLlc1(ref,fb); mode = 0;}
    (junction 50) -> (junction 51) [commented out]
    (junction 51) -> (junction 52) [commented out] : [loop_en == false]
    (junction 51) -> (junction 53) [commented out] : {loop_en = false}
    (junction 52) -> (junction 54) [commented out] : {loop_en = true}
    (junction 53) -> (junction 54) [commented out]
  state SSvoltage [function] [commented out]
  state ON_MODE
    entry:
    %%%%%%%%%%%
    during:
    %%%%%%%%%%%
    exit:
  state FAULT_LATCH
  state FAULT_RECOVERY
  (default) -> OFF_MODE
  OFF_MODE -> STARTUP_MODE : [pfc_ok == 1]
  STARTUP_MODE -> OFF_MODE [order 1] : [pfc_ok == 0]
  ON_MODE -> OFF_MODE [order 3] : [pfc_ok == 0]
  STARTUP_MODE -> ON_MODE [order 2] : [1]%softstart flag SoftStart_OK%
  ON_MODE -> FAULT_LATCH [order 1] : [0]
  ON_MODE -> FAULT_RECOVERY [order 2] : [0]
  data: ref_calib function_input double; fb function_input double; diff local double; pfc_ok input; llc_on output =0; SoftStart_OK local [0..1] =0; VBAT_Value input; RegulationPoint input; VBAT_Ref_adjusted output double =0
